simulink model "MassSpringDamperModel"  (R2023b)
settings: Solver=VariableStepAuto  StartTime=0.0  StopTime=10.0  RelTol=1e-3
settings Model: Creator=20181234  LastModifiedBy=20181234

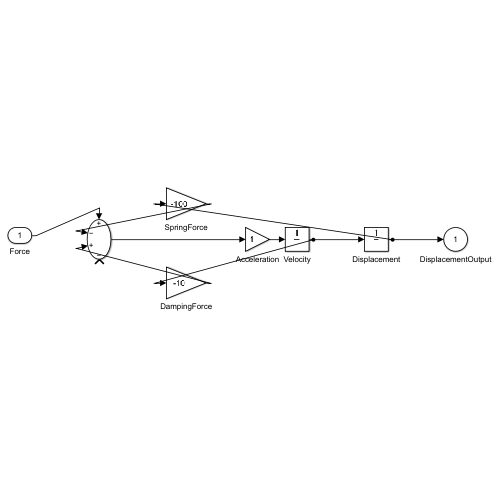
[thumbnail: Simulink's stored preview of the top-level diagram]
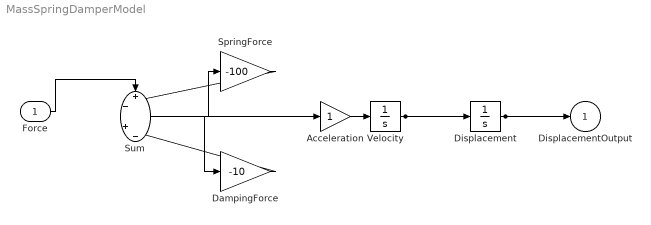
== system MassSpringDamperModel ==
  Force : Inport
  Acceleration : Gain
  DampingForce : Gain  Gain=-10
  Displacement : Integrator
  SpringForce : Gain  Gain=-100
  Sum : Sum  Inputs=+-+-
  Velocity : Integrator
  DisplacementOutput : Outport
  wires:
  Force/1 -> Sum/1
  Displacement/1 -> SpringForce/1, DisplacementOutput/1
  SpringForce/1 -> Sum/2
  Velocity/1 -> DampingForce/1, Displacement/1
  DampingForce/1 -> Sum/3
  Sum/1 -> Acceleration/1
  Acceleration/1 -> Velocity/1
